simulink model "RS232_controller"  (Simulink 7.4)
settings: Solver=FixedStepDiscrete  StartTime=0.0  StopTime=0.1  RelTol=1e-3
settings Model: Creator=robert  LastModifiedBy=roczit00

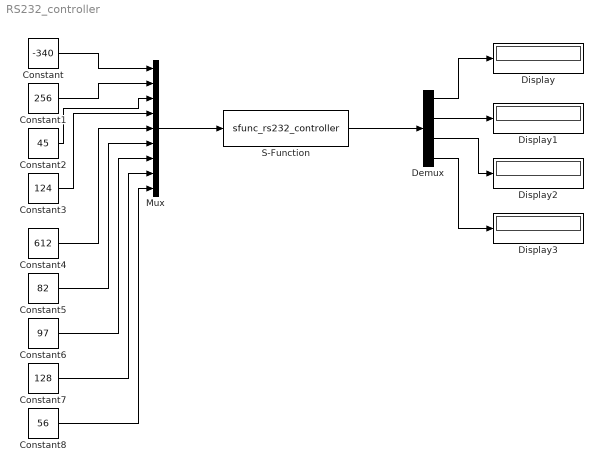
== system RS232_controller ==
  Constant : Constant  Value=-340  OutDataType=fixdt(1, 16)  OutScaling=2^0
  Constant1 : Constant  Value=256  OutDataType=fixdt(1, 16)  OutScaling=2^0
  Constant2 : Constant  Value=45  OutDataType=fixdt(1, 16)  OutScaling=2^0
  Constant3 : Constant  Value=124  OutDataType=fixdt(1, 16)  OutScaling=2^0
  Constant4 : Constant  Value=612  OutDataType=fixdt(1, 16)  OutScaling=2^0
  Constant5 : Constant  Value=82  OutDataType=fixdt(1, 16)  OutScaling=2^0
  Constant6 : Constant  Value=97  OutDataType=fixdt(1, 16)  OutScaling=2^0
  Constant7 : Constant  Value=128  OutDataType=fixdt(1, 16)  OutScaling=2^0
  Constant8 : Constant  Value=56  OutDataType=fixdt(1, 16)  OutScaling=2^0
  Demux : Demux
  Display{,1..3} (4 alike) : Display
  Mux : Mux  Inputs=9
  S-Function : S-Function  FunctionName=sfunc_rs232_controller  Parameters=Config  EnableBusSupport=off  mask{comport=0}
      mask prompts: comport "COM-Port (name):"
      mask init:
      | Config.COMPort = comport;
  wires:
  Mux/1 -> S-Function/1
  S-Function/1 -> Demux/1
  Demux/4 -> Display3/1
  Demux/3 -> Display2/1
  Demux/2 -> Display1/1
  Demux/1 -> Display/1
  Constant/1 -> Mux/1
  Constant1/1 -> Mux/2
  Constant2/1 -> Mux/3
  Constant3/1 -> Mux/4
  Constant4/1 -> Mux/5
  Constant5/1 -> Mux/6
  Constant6/1 -> Mux/7
  Constant7/1 -> Mux/8
  Constant8/1 -> Mux/9
